simulink model "OO_mode"  (R2020a)
settings: Solver=FixedStepAuto  StartTime=0.0  StopTime=10.0  FixedStep=1e-3  RelTol=1e-3  EnableMultiTasking=on
settings Model: ExtModeTrigDuration=5  Creator=zhanz173  LastModifiedBy=zhanz173
settings OptimizationCC: EnhancedBackFolding=on  PassReuseOutputArgsAs=Individual arguments  ZeroExternalMemoryAtStartup=off  ZeroInternalMemoryAtStartup=off  MaxStackSize=64  OptimizeBlockOrder=speed  DifferentSizesBufferReuse=on  OptimizationCustomize=off  EfficientTunableParamExpr=on
settings DebuggingCC: ParameterTunabilityLossMsg=error
settings HardwareCC: ProdBitPerPointer=32  ProdBitPerSizeT=32  ProdBitPerPtrDiffT=32  ProdLargestAtomicInteger=Long  ProdLargestAtomicFloat=Double  ProdWordSize=32  ProdHWDeviceType=ARM Compatible->ARM Cortex  TargetBitPerPointer=64  TargetBitPerSizeT=64  TargetBitPerPtrDiffT=64  TargetLongLongMode=on  TargetIntDivRoundTo=Zero  TargetEndianess=LittleEndian  TargetWordSize=64  TargetHWDeviceType=Custom Processor->MATLAB Host Computer  ProdEqTarget=off
settings SFSimCC: MATLABDynamicMemAlloc=off
settings RTWCC: SystemTargetFile=ert.tlc  HardwareBoard=NXP FRDM-K64F  TemplateMakefile=ert_default_tmf  Toolchain=GNU Tools for ARM Embedded Processors
settings CodeAppCC: ForceParamTrailComments=on  IgnoreCustomStorageClasses=off  OperatorAnnotations=on  SimulinkDataObjDesc=on  SFDataObjDesc=on  InsertBlockDesc=on

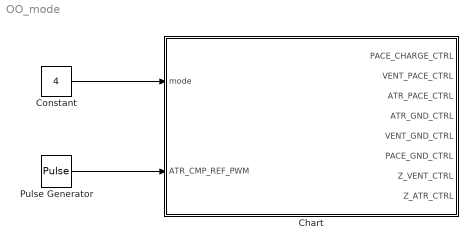
== system OO_mode ==
  Chart : Stateflow chart  TreatAsAtomicUnit=on
  Constant : Constant  Value=4
  Pulse Generator : DiscretePulseGenerator  PulseType=Time based  Period=10  PulseWidth=5
  wires:
  Pulse Generator/1 -> Chart/2(ATR_CMP_REF_PWM)
  Constant/1 -> Chart/1(mode)

== stateflow chart OO_mode/Chart ==
  state CHARGING
    entry:
    PACE_CHARGE_CTRL = 1
  state IDLE
    entry:
    ATR_PACE_CTRL = 0
    VENT_PACE_CTRL = 0
    Z_VENT_CTRL = 1;
    Z_ATR_CTRL = 1;
  state DELAY
  state Select_mode
    entry:
    VENT_GND_CTRL = 0
    ATR_GND_CTRL = 0
  state Atrial_Pacing
    entry:
    ATR_PACE_CTRL = 1
    VENT_PACE_CTRL = 0
    PACE_GND_CTRL = 1;
    Z_VENT_CTRL = 0;
    Z_ATR_CTRL = 0;
  state No_Pacing
    entry:
    ATR_PACE_CTRL = 0
    VENT_PACE_CTRL = 0
  state VVI
    entry:
  state AAI
    entry:
  state Ventricular_Pacing
    entry:
    ATR_PACE_CTRL = 0
    VENT_PACE_CTRL = 1
    PACE_GND_CTRL = 1;
    Z_VENT_CTRL = 0;
    Z_ATR_CTRL = 0;
  state Discharging
    entry:
    VENT_GND_CTRL = 1
    ATR_GND_CTRL = 1
  (default) -> IDLE
  Discharging -> IDLE
  IDLE -> CHARGING
  CHARGING -> DELAY
  VVI -> DELAY [order 1] : [VENT_RECT_SIGNAL == 1]
  AAI -> DELAY [order 2] : [ATR_RECT_SIGNAL == 1]
  DELAY -> Select_mode : after(10,msec)
  Select_mode -> VVI [order 5] : [mode == 4]
  Select_mode -> AAI [order 4] : [mode == 3]
  Select_mode -> Atrial_Pacing [order 1] : [mode == 1]
  Select_mode -> Ventricular_Pacing [order 2] : [mode == 2]
  Select_mode -> No_Pacing [order 3] : [mode == 5]
  AAI -> Atrial_Pacing [order 1] : [ATR_RECT_SIGNAL == 0]
  VVI -> Ventricular_Pacing [order 2] : [VENT_RECT_SIGNAL == 0]
  No_Pacing -> Discharging
  Atrial_Pacing -> Discharging
  Ventricular_Pacing -> Discharging
  data: PACE_CHARGE_CTRL output; VENT_PACE_CTRL output; ATR_PACE_CTRL output; ATR_GND_CTRL output; VENT_GND_CTRL output; PACE_GND_CTRL output; mode input; Z_VENT_CTRL output; Z_ATR_CTRL output; ATR_CMP_REF_PWM input
